simulink model "c28035pmsmfoc_cla"  (R2021b)
settings: Solver=FixedStepDiscrete  StartTime=0.0  StopTime=inf  RelTol=1e-3  EnableMultiTasking=on
PreLoadFcn:
  | c28035pmsmfoc_data_cla;
model workspace (MAT data in the model file):
  encoderResolution = 2000
  hallOffset = '0.5'
  indexOffset = 850
  polePairs = '4'
values from neighbouring files (symbols this model uses):
  Hall_position_offset = 0.57    [c28027pmsmfoc_data.m]    (also in c28035pmsmfoc_data.m; c28035pmsmfoc_data_cla.m; c28069pmsmfoc_data.m)
  PWM_Counter_Period = CPU_frequency/PWM_frequency/2    (= 1500)    [c28027pmsmfoc_data.m]    (also in c28035pmsmfoc_data.m; c28035pmsmfoc_data_cla.m = 2500; c28069pmsmfoc_data.m = 2250)
  Speed_per_unit_scaler = 1200    [c28027pmsmfoc_data.m]    (also in c28035pmsmfoc_data.m; c28035pmsmfoc_data_cla.m = 600; c28069pmsmfoc_data.m)
  Speed_rpm_scaler = 60*CPU_frequency/Pole_pairs/2    (= 450000000)    [c28027pmsmfoc_data.m]    (also in c28035pmsmfoc_data.m; c28035pmsmfoc_data_cla.m; c28069pmsmfoc_data.m = 675000000)
undefined symbols (not defined in the file or in its folder): codertarget, Down, GPTRIP1SEL, GPTRIP2SEL, TZ1, TZ2, Up
libraries: idelinklib_common x16, tiiqmathlib x7, hall_sensor_lib x7, c2802xlib x6, simulink x3, c2803xlib x2, etargetslib x2, demo_controls x1, c2806xlib x1, c280xlib x1, c2000lib x1
(part 3 of 3)

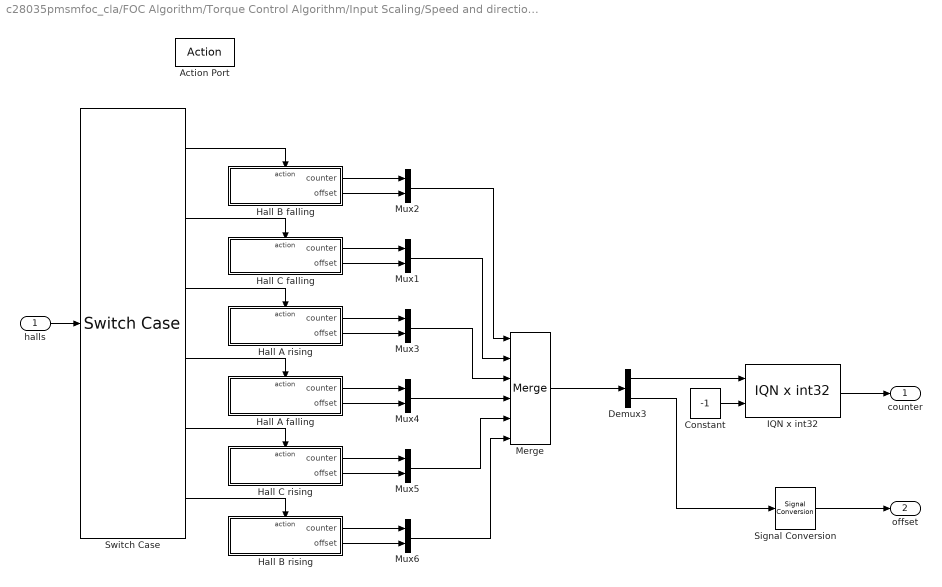
== system c28035pmsmfoc_cla/FOC Algorithm/Torque Control Algorithm/Input Scaling/Speed and direction are valid Use speed to extrapolate position/Extract Position from Halls/Direction 1 Provides offset and counter values ==
  halls : Inport
  Action Port : ActionPort  ActionPortLabel=if(u1 ~= 0)
  Constant : Constant  Value=-1  OutDataTypeStr=int32
  Demux3 : Demux  Outputs=2
  Hall A falling : Subsystem  TreatAsAtomicUnit=on
  Hall A rising : Subsystem  TreatAsAtomicUnit=on
  Hall B falling : Subsystem  TreatAsAtomicUnit=on
  Hall B rising : Subsystem  TreatAsAtomicUnit=on
  Hall C falling : Subsystem  TreatAsAtomicUnit=on
  Hall C rising : Subsystem  TreatAsAtomicUnit=on
  IQN x int32 : tiiqmathlib/IQN x int32
      settings: SourceProductBaseCode=TIC2000
  Merge : Merge  Inputs=6
  Mux{1..6} (6 alike) : Mux  Inputs=2
  Signal Conversion : SignalConversion  OverrideOpt=on
  Switch Case : SwitchCase  CaseConditions={1,2,3,4,5,6}  ShowDefaultCase=off
  counter : Outport
  offset : Outport  Port=2
  wires:
  Hall B falling/1(counter) -> Mux2/1
  Hall B falling/2(offset) -> Mux2/2
  Hall C falling/1(counter) -> Mux1/1
  Hall C falling/2(offset) -> Mux1/2
  Hall A rising/1(counter) -> Mux3/1
  Hall A rising/2(offset) -> Mux3/2
  Hall A falling/1(counter) -> Mux4/1
  Hall A falling/2(offset) -> Mux4/2
  Hall C rising/1(counter) -> Mux5/1
  Hall C rising/2(offset) -> Mux5/2
  Hall B rising/1(counter) -> Mux6/1
  Hall B rising/2(offset) -> Mux6/2
  Mux2/1 -> Merge/1
  Mux1/1 -> Merge/2
  Mux3/1 -> Merge/3
  Mux4/1 -> Merge/4
  Mux5/1 -> Merge/5
  Mux6/1 -> Merge/6
  Merge/1 -> Demux3/1
  Demux3/1 -> IQN x int32/1
  Demux3/2 -> Signal Conversion/1
  IQN x int32/1 -> counter/1
  Constant/1 -> IQN x int32/2
  halls/1 -> Switch Case/1
  Switch Case/2 -> Hall C falling/Action
  Switch Case/5 -> Hall C rising/Action
  Switch Case/6 -> Hall B rising/Action
  Switch Case/1 -> Hall B falling/Action
  Switch Case/3 -> Hall A rising/Action
  Switch Case/4 -> Hall A falling/Action
  Signal Conversion/1 -> offset/1

== system c28035pmsmfoc_cla/FOC Algorithm/Torque Control Algorithm/Generating Space Vectors/Generating Raw Space Vectors/SVGen/Sectors 1//2//3/Sector 1 ==
  Vb* : Inport
  Vc* : Inport  Port=2
  Action Port : ActionPort  ActionPortLabel=else
  Add : Sum  Inputs=--+
  Add1 : Sum
  Add2 : Sum
  Constant : Constant  OutDataTypeStr=Inherit: Inherit via back propagation
  Constant1 : Constant  Value=0.5  OutDataTypeStr=Inherit: Inherit via back propagation
  Product : Product
  Signal Conversion : SignalConversion  OverrideOpt=off
  Signal Conversion1 : SignalConversion  OverrideOpt=off
  Ta* : Outport
  Tb* : Outport  Port=2
  Tc* : Outport  Port=3
  wires:
  Add1/1 -> Tc*/1
  Vc*/1 -> Add2/1, Add/2
  Vb*/1 -> Add1/2, Add/1
  Add2/1 -> Signal Conversion1/1, Add1/1
  Constant1/1 -> Product/2
  Add/1 -> Product/1
  Product/1 -> Signal Conversion/1, Add2/2
  Constant/1 -> Add/3
  Signal Conversion/1 -> Tb*/1
  Signal Conversion1/1 -> Ta*/1

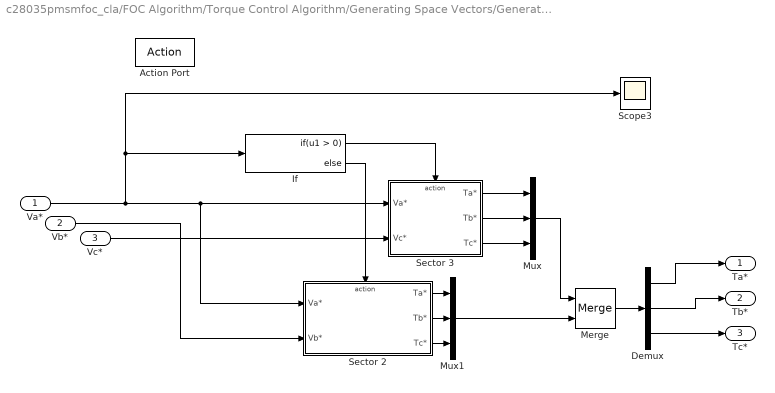
== system c28035pmsmfoc_cla/FOC Algorithm/Torque Control Algorithm/Generating Space Vectors/Generating Raw Space Vectors/SVGen/Sectors 1//2//3/Sector 2 and 3 ==
  Va* : Inport
  Vb* : Inport  Port=2
  Vc* : Inport  Port=3
  Action Port : ActionPort  ActionPortLabel=if(u1 > 0)
  Demux : Demux  Outputs=3
  If : If
  Merge : Merge
  Mux : Mux  Inputs=3
  Mux1 : Mux  Inputs=3
  Scope3 : Scope
  Sector 2 : Subsystem  TreatAsAtomicUnit=on
  Sector 3 : Subsystem  TreatAsAtomicUnit=on
  Ta* : Outport
  Tb* : Outport  Port=2
  Tc* : Outport  Port=3
  wires:
  Va*/1 -> Sector 2/1(Va*), Sector 3/1(Va*), If/1, Scope3/1
  Vb*/1 -> Sector 2/2(Vb*)
  If/1 -> Sector 3/Action
  If/2 -> Sector 2/Action
  Vc*/1 -> Sector 3/2(Vc*)
  Sector 3/1(Ta*) -> Mux/1
  Sector 3/2(Tb*) -> Mux/2
  Sector 3/3(Tc*) -> Mux/3
  Sector 2/1(Ta*) -> Mux1/1
  Sector 2/2(Tb*) -> Mux1/2
  Sector 2/3(Tc*) -> Mux1/3
  Mux/1 -> Merge/1
  Mux1/1 -> Merge/2
  Merge/1 -> Demux/1
  Demux/1 -> Ta*/1
  Demux/2 -> Tb*/1
  Demux/3 -> Tc*/1

== system c28035pmsmfoc_cla/FOC Algorithm/Torque Control Algorithm/Generating Space Vectors/Generating Raw Space Vectors/SVGen/Sectors 4//5//6/Sector 4 and 5 ==
  Va* : Inport
  Vb* : Inport  Port=2
  Vc* : Inport  Port=3
  Action Port : ActionPort  ActionPortLabel=else
  Demux : Demux  Outputs=3
  If : If
  Merge : Merge
  Mux : Mux  Inputs=3
  Mux1 : Mux  Inputs=3
  Sector 4 : Subsystem  TreatAsAtomicUnit=on
  Sector 5 : Subsystem  TreatAsAtomicUnit=on
  Ta* : Outport
  Tb* : Outport  Port=2
  Tc* : Outport  Port=3
  wires:
  Va*/1 -> If/1, Sector 4/1(Va*), Sector 5/1(Va*)
  Demux/3 -> Tc*/1
  Demux/2 -> Tb*/1
  Demux/1 -> Ta*/1
  Merge/1 -> Demux/1
  Mux1/1 -> Merge/2
  Mux/1 -> Merge/1
  Sector 4/3(Tc*) -> Mux1/3
  Sector 4/2(Tb*) -> Mux1/2
  Sector 4/1(Ta*) -> Mux1/1
  Sector 5/3(Tc*) -> Mux/3
  Sector 5/2(Tb*) -> Mux/2
  Sector 5/1(Ta*) -> Mux/1
  Vc*/1 -> Sector 4/2(Vc*)
  Vb*/1 -> Sector 5/2(Vb*)
  If/2 -> Sector 4/Action
  If/1 -> Sector 5/Action

== system c28035pmsmfoc_cla/FOC Algorithm/Torque Control Algorithm/Generating Space Vectors/Generating Raw Space Vectors/SVGen/Sectors 4//5//6/Sector 6 ==
  Vb* : Inport
  Vc* : Inport  Port=2
  Action Port : ActionPort  ActionPortLabel=if(u1 > 0)
  Add : Sum  Inputs=+++
  Add1 : Sum  Inputs=+-
  Add2 : Sum  Inputs=-+
  Constant : Constant  OutDataTypeStr=Inherit: Inherit via back propagation
  Constant1 : Constant  Value=0.5  OutDataTypeStr=Inherit: Inherit via back propagation
  Product : Product
  Signal Conversion1 : SignalConversion  OverrideOpt=off
  Signal Conversion2 : SignalConversion  OverrideOpt=off
  Ta* : Outport
  Tb* : Outport  Port=2
  Tc* : Outport  Port=3
  wires:
  Add1/1 -> Tb*/1
  Add2/1 -> Add1/1, Signal Conversion2/1
  Constant1/1 -> Product/2
  Add/1 -> Product/1
  Product/1 -> Add2/2, Signal Conversion1/1
  Constant/1 -> Add/3
  Vc*/1 -> Add1/2, Add/2
  Vb*/1 -> Add2/1, Add/1
  Signal Conversion2/1 -> Ta*/1
  Signal Conversion1/1 -> Tc*/1

== system c28035pmsmfoc_cla/FOC Algorithm/Torque Control Algorithm/Generating Space Vectors/Generating Raw Space Vectors/control/PID Controller/UD_REG3 ==
  up_reg3 : Inport
  PrevOut : Inport  Port=2
  Constant : Constant  Value=derivativeGain  OutDataTypeStr=Inherit: Inherit via back propagation
  Product : Product  OutDataTypeStr=Inherit: Same as first input
  Sum2 : Sum  Inputs=+-
  Out1 : Outport
  wires:
  Constant/1 -> Product/1
  Product/1 -> Out1/1
  Sum2/1 -> Product/2
  PrevOut/1 -> Sum2/2
  up_reg3/1 -> Sum2/1

== system c28035pmsmfoc_cla/FOC Algorithm/Torque Control Algorithm/Generating Space Vectors/Generating Raw Space Vectors/control/PID Controller/UI_REG3 ==
  OLD_UI_REG3 : Inport
  up_reg3 : Inport  Port=2
  saterr_reg3 : Inport  Port=3
  Constant : Constant  Value=integralGain  OutDataTypeStr=Inherit: Inherit via back propagation
  Constant1 : Constant  Value=correctionGain  OutDataTypeStr=Inherit: Inherit via back propagation
  Product : Product  OutDataTypeStr=Inherit: Same as first input
  Product1 : Product  OutDataTypeStr=Inherit: Same as first input
  Sum1 : Sum  Inputs=+++
  UI_REG1 : Outport
  wires:
  Constant1/1 -> Product1/1
  saterr_reg3/1 -> Product1/2
  Constant/1 -> Product/1
  up_reg3/1 -> Product/2
  Sum1/1 -> UI_REG1/1
  Product1/1 -> Sum1/3
  Product/1 -> Sum1/2
  OLD_UI_REG3/1 -> Sum1/1

== system c28035pmsmfoc_cla/FOC Algorithm/Torque Control Algorithm/Generating Space Vectors/Generating Raw Space Vectors/control/PID Controller1/UD_REG3 ==
  up_reg3 : Inport
  PrevOut : Inport  Port=2
  Constant : Constant  Value=derivativeGain  OutDataTypeStr=Inherit: Inherit via back propagation
  Product : Product  OutDataTypeStr=Inherit: Same as first input
  Sum2 : Sum  Inputs=+-
  Out1 : Outport
  wires:
  Constant/1 -> Product/1
  Product/1 -> Out1/1
  Sum2/1 -> Product/2
  PrevOut/1 -> Sum2/2
  up_reg3/1 -> Sum2/1

== system c28035pmsmfoc_cla/FOC Algorithm/Torque Control Algorithm/Generating Space Vectors/Generating Raw Space Vectors/control/PID Controller1/UI_REG3 ==
  OLD_UI_REG3 : Inport
  up_reg3 : Inport  Port=2
  saterr_reg3 : Inport  Port=3
  Constant : Constant  Value=integralGain  OutDataTypeStr=Inherit: Inherit via back propagation
  Constant1 : Constant  Value=correctionGain  OutDataTypeStr=Inherit: Inherit via back propagation
  Product : Product  OutDataTypeStr=Inherit: Same as first input
  Product1 : Product  OutDataTypeStr=Inherit: Same as first input
  Sum1 : Sum  Inputs=+++
  UI_REG1 : Outport
  wires:
  Constant1/1 -> Product1/1
  saterr_reg3/1 -> Product1/2
  Constant/1 -> Product/1
  up_reg3/1 -> Product/2
  Sum1/1 -> UI_REG1/1
  Product1/1 -> Sum1/3
  Product/1 -> Sum1/2
  OLD_UI_REG3/1 -> Sum1/1

== system c28035pmsmfoc_cla/FOC Algorithm/Torque Control Algorithm/Input Scaling/Speed and direction are valid Use speed to extrapolate position/Extract Position from Halls/Direction 0 Provides offset and counter values/Hall A falling ==
  Action Port : ActionPort  ActionPortLabel=case [ 2 ]:
  Constant : Constant  Value=1/2  OutDataTypeStr=fixdt(1,32,17)
  Data Type Conversion1 : DataTypeConversion  OutDataTypeStr=fixdt(1,32,17)  ConvertRealWorld=Stored Integer (SI)
  ECap1Regs.TSCTR1 : idelinklib_common/Memory Copy  copyFrom=Specified source code symbol  copyFromAddressSource=Specify via dialog  copyFromAddress=hex2dec('00001000')  copyFromSrcCode=&ECap1Regs.TSCTR  dataTypeFrom=uint32  dataDimensionFrom=1  useOffsetFrom=off  offsetFromSrc=Specify via dialog  offsetFrom=0  strideFrom=1  copyTo=Output port  copyToAddressSource=Specify via dialog  copyToAddress=hex2dec('00002000')  copyToSrcCode=myVariableDst  dataTypeTo=uint32  useOffsetTo=off  offsetToSrc=Specify via dialog  offsetTo=0  strideTo=1  sampleTime=-1  useInitValue=off  initValueSrc=Specify constant value  initValue=1  initValueSrcCode=myInitValueVariable  useAsMask=off  maskOperator=bitwise AND  useTermValue=off  termValue=1  isRealtimeEnabled=off  emitCCBeforeWrite=off  CCBeforeWrite=/* Custom Code Before Write*/  emitCCAfterWrite=off  CCAfterWrite=/* Custom Code After Write*/  useDMACopy=off  enableBlockingMode=off
      settings: SourceProductBaseCode=ME
  counter : Outport
  offset : Outport  Port=2
  wires:
  Constant/1 -> offset/1
  ECap1Regs.TSCTR1/1 -> Data Type Conversion1/1
  Data Type Conversion1/1 -> counter/1

== system c28035pmsmfoc_cla/FOC Algorithm/Torque Control Algorithm/Input Scaling/Speed and direction are valid Use speed to extrapolate position/Extract Position from Halls/Direction 0 Provides offset and counter values/Hall A rising ==
  Action Port : ActionPort  ActionPortLabel=case [ 5 ]:
  Constant : Constant  Value=0  OutDataTypeStr=fixdt(1,32,17)
  Data Type Conversion1 : DataTypeConversion  OutDataTypeStr=fixdt(1,32,17)  ConvertRealWorld=Stored Integer (SI)
  ECap1Regs.TSCTR1 : idelinklib_common/Memory Copy  copyFrom=Specified source code symbol  copyFromAddressSource=Specify via dialog  copyFromAddress=hex2dec('00001000')  copyFromSrcCode=&ECap1Regs.TSCTR  dataTypeFrom=uint32  dataDimensionFrom=1  useOffsetFrom=off  offsetFromSrc=Specify via dialog  offsetFrom=0  strideFrom=1  copyTo=Output port  copyToAddressSource=Specify via dialog  copyToAddress=hex2dec('00002000')  copyToSrcCode=myVariableDst  dataTypeTo=uint32  useOffsetTo=off  offsetToSrc=Specify via dialog  offsetTo=0  strideTo=1  sampleTime=-1  useInitValue=off  initValueSrc=Specify constant value  initValue=1  initValueSrcCode=myInitValueVariable  useAsMask=off  maskOperator=bitwise AND  useTermValue=off  termValue=1  isRealtimeEnabled=off  emitCCBeforeWrite=off  CCBeforeWrite=/* Custom Code Before Write*/  emitCCAfterWrite=off  CCAfterWrite=/* Custom Code After Write*/  useDMACopy=off  enableBlockingMode=off
      settings: SourceProductBaseCode=ME
  counter : Outport
  offset : Outport  Port=2
  wires:
  Constant/1 -> offset/1
  ECap1Regs.TSCTR1/1 -> Data Type Conversion1/1
  Data Type Conversion1/1 -> counter/1

== system c28035pmsmfoc_cla/FOC Algorithm/Torque Control Algorithm/Input Scaling/Speed and direction are valid Use speed to extrapolate position/Extract Position from Halls/Direction 0 Provides offset and counter values/Hall B falling ==
  Action Port : ActionPort  ActionPortLabel=case [ 4 ]:
  Add : Sum  Inputs=-+  OutDataTypeStr=Inherit: Same as first input
  Constant : Constant  Value=5/6  OutDataTypeStr=fixdt(1,32,17)
  Data Store Read : DataStoreRead  DataStoreName=ECap1_counter_XINT1_latch  IndexOptions=Index vector (dialog)  Indices=1  OutputSizes=1
  Data Type Conversion1 : DataTypeConversion  OutDataTypeStr=fixdt(1,32,17)  ConvertRealWorld=Stored Integer (SI)
  ECap1Regs.TSCTR : idelinklib_common/Memory Copy  copyFrom=Specified source code symbol  copyFromAddressSource=Specify via dialog  copyFromAddress=hex2dec('00001000')  copyFromSrcCode=&ECap1Regs.TSCTR  dataTypeFrom=uint32  dataDimensionFrom=1  useOffsetFrom=off  offsetFromSrc=Specify via dialog  offsetFrom=0  strideFrom=1  copyTo=Output port  copyToAddressSource=Specify via dialog  copyToAddress=hex2dec('00002000')  copyToSrcCode=myVariableDst  dataTypeTo=uint32  useOffsetTo=off  offsetToSrc=Specify via dialog  offsetTo=0  strideTo=1  sampleTime=-1  useInitValue=off  initValueSrc=Specify constant value  initValue=1  initValueSrcCode=myInitValueVariable  useAsMask=off  maskOperator=bitwise AND  useTermValue=off  termValue=1  isRealtimeEnabled=off  emitCCBeforeWrite=off  CCBeforeWrite=/* Custom Code Before Write*/  emitCCAfterWrite=off  CCAfterWrite=/* Custom Code After Write*/  useDMACopy=off  enableBlockingMode=off
      settings: SourceProductBaseCode=ME
  counter : Outport
  offset : Outport  Port=2
  wires:
  Constant/1 -> offset/1
  Data Type Conversion1/1 -> counter/1
  Data Store Read/1 -> Add/1
  ECap1Regs.TSCTR/1 -> Add/2
  Add/1 -> Data Type Conversion1/1

== system c28035pmsmfoc_cla/FOC Algorithm/Torque Control Algorithm/Input Scaling/Speed and direction are valid Use speed to extrapolate position/Extract Position from Halls/Direction 0 Provides offset and counter values/Hall B rising ==
  Action Port : ActionPort  ActionPortLabel=case [ 3 ]:
  Add : Sum  Inputs=-+  OutDataTypeStr=Inherit: Same as first input
  Constant : Constant  Value=2/6  OutDataTypeStr=fixdt(1,32,17)
  Data Store Read : DataStoreRead  DataStoreName=ECap1_counter_XINT1_latch  IndexOptions=Index vector (dialog)  Indices=1  OutputSizes=1
  Data Type Conversion1 : DataTypeConversion  OutDataTypeStr=fixdt(1,32,17)  ConvertRealWorld=Stored Integer (SI)
  ECap1Regs.TSCTR : idelinklib_common/Memory Copy  copyFrom=Specified source code symbol  copyFromAddressSource=Specify via dialog  copyFromAddress=hex2dec('00001000')  copyFromSrcCode=&ECap1Regs.TSCTR  dataTypeFrom=uint32  dataDimensionFrom=1  useOffsetFrom=off  offsetFromSrc=Specify via dialog  offsetFrom=0  strideFrom=1  copyTo=Output port  copyToAddressSource=Specify via dialog  copyToAddress=hex2dec('00002000')  copyToSrcCode=myVariableDst  dataTypeTo=uint32  useOffsetTo=off  offsetToSrc=Specify via dialog  offsetTo=0  strideTo=1  sampleTime=-1  useInitValue=off  initValueSrc=Specify constant value  initValue=1  initValueSrcCode=myInitValueVariable  useAsMask=off  maskOperator=bitwise AND  useTermValue=off  termValue=1  isRealtimeEnabled=off  emitCCBeforeWrite=off  CCBeforeWrite=/* Custom Code Before Write*/  emitCCAfterWrite=off  CCAfterWrite=/* Custom Code After Write*/  useDMACopy=off  enableBlockingMode=off
      settings: SourceProductBaseCode=ME
  counter : Outport
  offset : Outport  Port=2
  wires:
  Constant/1 -> offset/1
  Data Type Conversion1/1 -> counter/1
  Data Store Read/1 -> Add/1
  ECap1Regs.TSCTR/1 -> Add/2
  Add/1 -> Data Type Conversion1/1

== system c28035pmsmfoc_cla/FOC Algorithm/Torque Control Algorithm/Input Scaling/Speed and direction are valid Use speed to extrapolate position/Extract Position from Halls/Direction 0 Provides offset and counter values/Hall C falling ==
  Action Port : ActionPort  ActionPortLabel=case [ 1 ]:
  Add : Sum  Inputs=-+  OutDataTypeStr=Inherit: Same as first input
  Constant : Constant  Value=1/6  OutDataTypeStr=fixdt(1,32,17)
  Data Store Read : DataStoreRead  DataStoreName=ECap1_counter_XINT2_latch  IndexOptions=Index vector (dialog)  Indices=1  OutputSizes=1
  Data Type Conversion1 : DataTypeConversion  OutDataTypeStr=fixdt(1,32,17)  ConvertRealWorld=Stored Integer (SI)
  ECap1Regs.TSCTR : idelinklib_common/Memory Copy  copyFrom=Specified source code symbol  copyFromAddressSource=Specify via dialog  copyFromAddress=hex2dec('00001000')  copyFromSrcCode=&ECap1Regs.TSCTR  dataTypeFrom=uint32  dataDimensionFrom=1  useOffsetFrom=off  offsetFromSrc=Specify via dialog  offsetFrom=0  strideFrom=1  copyTo=Output port  copyToAddressSource=Specify via dialog  copyToAddress=hex2dec('00002000')  copyToSrcCode=myVariableDst  dataTypeTo=uint32  useOffsetTo=off  offsetToSrc=Specify via dialog  offsetTo=0  strideTo=1  sampleTime=-1  useInitValue=off  initValueSrc=Specify constant value  initValue=1  initValueSrcCode=myInitValueVariable  useAsMask=off  maskOperator=bitwise AND  useTermValue=off  termValue=1  isRealtimeEnabled=off  emitCCBeforeWrite=off  CCBeforeWrite=/* Custom Code Before Write*/  emitCCAfterWrite=off  CCAfterWrite=/* Custom Code After Write*/  useDMACopy=off  enableBlockingMode=off
      settings: SourceProductBaseCode=ME
  counter : Outport
  offset : Outport  Port=2
  wires:
  Constant/1 -> offset/1
  Data Type Conversion1/1 -> counter/1
  Data Store Read/1 -> Add/1
  ECap1Regs.TSCTR/1 -> Add/2
  Add/1 -> Data Type Conversion1/1

== system c28035pmsmfoc_cla/FOC Algorithm/Torque Control Algorithm/Input Scaling/Speed and direction are valid Use speed to extrapolate position/Extract Position from Halls/Direction 0 Provides offset and counter values/Hall C rising ==
  Action Port : ActionPort  ActionPortLabel=case [ 6 ]:
  Add : Sum  Inputs=-+  OutDataTypeStr=Inherit: Same as first input
  Constant : Constant  Value=2/3  OutDataTypeStr=fixdt(1,32,17)
  Data Store Read : DataStoreRead  DataStoreName=ECap1_counter_XINT2_latch  IndexOptions=Index vector (dialog)  Indices=1  OutputSizes=1
  Data Type Conversion1 : DataTypeConversion  OutDataTypeStr=fixdt(1,32,17)  ConvertRealWorld=Stored Integer (SI)
  ECap1Regs.TSCTR : idelinklib_common/Memory Copy  copyFrom=Specified source code symbol  copyFromAddressSource=Specify via dialog  copyFromAddress=hex2dec('00001000')  copyFromSrcCode=&ECap1Regs.TSCTR  dataTypeFrom=uint32  dataDimensionFrom=1  useOffsetFrom=off  offsetFromSrc=Specify via dialog  offsetFrom=0  strideFrom=1  copyTo=Output port  copyToAddressSource=Specify via dialog  copyToAddress=hex2dec('00002000')  copyToSrcCode=myVariableDst  dataTypeTo=uint32  useOffsetTo=off  offsetToSrc=Specify via dialog  offsetTo=0  strideTo=1  sampleTime=-1  useInitValue=off  initValueSrc=Specify constant value  initValue=1  initValueSrcCode=myInitValueVariable  useAsMask=off  maskOperator=bitwise AND  useTermValue=off  termValue=1  isRealtimeEnabled=off  emitCCBeforeWrite=off  CCBeforeWrite=/* Custom Code Before Write*/  emitCCAfterWrite=off  CCAfterWrite=/* Custom Code After Write*/  useDMACopy=off  enableBlockingMode=off
      settings: SourceProductBaseCode=ME
  counter : Outport
  offset : Outport  Port=2
  wires:
  Constant/1 -> offset/1
  Data Type Conversion1/1 -> counter/1
  Data Store Read/1 -> Add/1
  ECap1Regs.TSCTR/1 -> Add/2
  Add/1 -> Data Type Conversion1/1

== system c28035pmsmfoc_cla/FOC Algorithm/Torque Control Algorithm/Input Scaling/Speed and direction are valid Use speed to extrapolate position/Extract Position from Halls/Direction 1 Provides offset and counter values/Hall A falling ==
  Action Port : ActionPort  ActionPortLabel=case [ 4 ]:
  Constant : Constant  OutDataTypeStr=fixdt(1,32,17)
  Data Type Conversion1 : DataTypeConversion  OutDataTypeStr=fixdt(1,32,17)  ConvertRealWorld=Stored Integer (SI)
  ECap1Regs.TSCTR1 : idelinklib_common/Memory Copy  copyFrom=Specified source code symbol  copyFromAddressSource=Specify via dialog  copyFromAddress=hex2dec('00001000')  copyFromSrcCode=&ECap1Regs.TSCTR  dataTypeFrom=uint32  dataDimensionFrom=1  useOffsetFrom=off  offsetFromSrc=Specify via dialog  offsetFrom=0  strideFrom=1  copyTo=Output port  copyToAddressSource=Specify via dialog  copyToAddress=hex2dec('00002000')  copyToSrcCode=myVariableDst  dataTypeTo=uint32  useOffsetTo=off  offsetToSrc=Specify via dialog  offsetTo=0  strideTo=1  sampleTime=-1  useInitValue=off  initValueSrc=Specify constant value  initValue=1  initValueSrcCode=myInitValueVariable  useAsMask=off  maskOperator=bitwise AND  useTermValue=off  termValue=1  isRealtimeEnabled=off  emitCCBeforeWrite=off  CCBeforeWrite=/* Custom Code Before Write*/  emitCCAfterWrite=off  CCAfterWrite=/* Custom Code After Write*/  useDMACopy=off  enableBlockingMode=off
      settings: SourceProductBaseCode=ME
  counter : Outport
  offset : Outport  Port=2
  wires:
  Data Type Conversion1/1 -> counter/1
  ECap1Regs.TSCTR1/1 -> Data Type Conversion1/1
  Constant/1 -> offset/1

== system c28035pmsmfoc_cla/FOC Algorithm/Torque Control Algorithm/Input Scaling/Speed and direction are valid Use speed to extrapolate position/Extract Position from Halls/Direction 1 Provides offset and counter values/Hall A rising ==
  Action Port : ActionPort  ActionPortLabel=case [ 3 ]:
  Constant : Constant  Value=1/2  OutDataTypeStr=fixdt(1,32,17)
  Data Type Conversion1 : DataTypeConversion  OutDataTypeStr=fixdt(1,32,17)  ConvertRealWorld=Stored Integer (SI)
  ECap1Regs.TSCTR1 : idelinklib_common/Memory Copy  copyFrom=Specified source code symbol  copyFromAddressSource=Specify via dialog  copyFromAddress=hex2dec('00001000')  copyFromSrcCode=&ECap1Regs.TSCTR  dataTypeFrom=uint32  dataDimensionFrom=1  useOffsetFrom=off  offsetFromSrc=Specify via dialog  offsetFrom=0  strideFrom=1  copyTo=Output port  copyToAddressSource=Specify via dialog  copyToAddress=hex2dec('00002000')  copyToSrcCode=myVariableDst  dataTypeTo=uint32  useOffsetTo=off  offsetToSrc=Specify via dialog  offsetTo=0  strideTo=1  sampleTime=-1  useInitValue=off  initValueSrc=Specify constant value  initValue=1  initValueSrcCode=myInitValueVariable  useAsMask=off  maskOperator=bitwise AND  useTermValue=off  termValue=1  isRealtimeEnabled=off  emitCCBeforeWrite=off  CCBeforeWrite=/* Custom Code Before Write*/  emitCCAfterWrite=off  CCAfterWrite=/* Custom Code After Write*/  useDMACopy=off  enableBlockingMode=off
      settings: SourceProductBaseCode=ME
  counter : Outport
  offset : Outport  Port=2
  wires:
  Data Type Conversion1/1 -> counter/1
  ECap1Regs.TSCTR1/1 -> Data Type Conversion1/1
  Constant/1 -> offset/1

== system c28035pmsmfoc_cla/FOC Algorithm/Torque Control Algorithm/Input Scaling/Speed and direction are valid Use speed to extrapolate position/Extract Position from Halls/Direction 1 Provides offset and counter values/Hall B falling ==
  Action Port : ActionPort  ActionPortLabel=case [ 1 ]:
  Add : Sum  Inputs=+-  OutDataTypeStr=Inherit: Same as first input
  Constant : Constant  Value=1/3  OutDataTypeStr=fixdt(1,32,17)
  Data Store Read : DataStoreRead  DataStoreName=ECap1_counter_XINT1_latch  IndexOptions=Index vector (dialog)  Indices=1  OutputSizes=1
  Data Type Conversion1 : DataTypeConversion  OutDataTypeStr=fixdt(1,32,17)  ConvertRealWorld=Stored Integer (SI)
  ECap1Regs.TSCTR : idelinklib_common/Memory Copy  copyFrom=Specified source code symbol  copyFromAddressSource=Specify via dialog  copyFromAddress=hex2dec('00001000')  copyFromSrcCode=&ECap1Regs.TSCTR  dataTypeFrom=uint32  dataDimensionFrom=1  useOffsetFrom=off  offsetFromSrc=Specify via dialog  offsetFrom=0  strideFrom=1  copyTo=Output port  copyToAddressSource=Specify via dialog  copyToAddress=hex2dec('00002000')  copyToSrcCode=myVariableDst  dataTypeTo=uint32  useOffsetTo=off  offsetToSrc=Specify via dialog  offsetTo=0  strideTo=1  sampleTime=-1  useInitValue=off  initValueSrc=Specify constant value  initValue=1  initValueSrcCode=myInitValueVariable  useAsMask=off  maskOperator=bitwise AND  useTermValue=off  termValue=1  isRealtimeEnabled=off  emitCCBeforeWrite=off  CCBeforeWrite=/* Custom Code Before Write*/  emitCCAfterWrite=off  CCAfterWrite=/* Custom Code After Write*/  useDMACopy=off  enableBlockingMode=off
      settings: SourceProductBaseCode=ME
  counter : Outport
  offset : Outport  Port=2
  wires:
  Data Type Conversion1/1 -> counter/1
  Constant/1 -> offset/1
  Add/1 -> Data Type Conversion1/1
  ECap1Regs.TSCTR/1 -> Add/1
  Data Store Read/1 -> Add/2

== system c28035pmsmfoc_cla/FOC Algorithm/Torque Control Algorithm/Input Scaling/Speed and direction are valid Use speed to extrapolate position/Extract Position from Halls/Direction 1 Provides offset and counter values/Hall B rising ==
  Action Port : ActionPort  ActionPortLabel=case [ 6 ]:
  Add : Sum  Inputs=-+  OutDataTypeStr=Inherit: Same as first input
  Constant : Constant  Value=5/6  OutDataTypeStr=fixdt(1,32,17)
  Data Store Read : DataStoreRead  DataStoreName=ECap1_counter_XINT1_latch  IndexOptions=Index vector (dialog)  Indices=1  OutputSizes=1
  Data Type Conversion2 : DataTypeConversion  OutDataTypeStr=fixdt(1,32,17)  ConvertRealWorld=Stored Integer (SI)
  ECap1Regs.TSCTR : idelinklib_common/Memory Copy  copyFrom=Specified source code symbol  copyFromAddressSource=Specify via dialog  copyFromAddress=hex2dec('00001000')  copyFromSrcCode=&ECap1Regs.TSCTR  dataTypeFrom=uint32  dataDimensionFrom=1  useOffsetFrom=off  offsetFromSrc=Specify via dialog  offsetFrom=0  strideFrom=1  copyTo=Output port  copyToAddressSource=Specify via dialog  copyToAddress=hex2dec('00002000')  copyToSrcCode=myVariableDst  dataTypeTo=uint32  useOffsetTo=off  offsetToSrc=Specify via dialog  offsetTo=0  strideTo=1  sampleTime=-1  useInitValue=off  initValueSrc=Specify constant value  initValue=1  initValueSrcCode=myInitValueVariable  useAsMask=off  maskOperator=bitwise AND  useTermValue=off  termValue=1  isRealtimeEnabled=off  emitCCBeforeWrite=off  CCBeforeWrite=/* Custom Code Before Write*/  emitCCAfterWrite=off  CCAfterWrite=/* Custom Code After Write*/  useDMACopy=off  enableBlockingMode=off
      settings: SourceProductBaseCode=ME
  counter : Outport
  offset : Outport  Port=2
  wires:
  Data Type Conversion2/1 -> counter/1
  Constant/1 -> offset/1
  Data Store Read/1 -> Add/1
  ECap1Regs.TSCTR/1 -> Add/2
  Add/1 -> Data Type Conversion2/1

== system c28035pmsmfoc_cla/FOC Algorithm/Torque Control Algorithm/Input Scaling/Speed and direction are valid Use speed to extrapolate position/Extract Position from Halls/Direction 1 Provides offset and counter values/Hall C falling ==
  Action Port : ActionPort  ActionPortLabel=case [ 2 ]:
  Add : Sum  Inputs=-+  OutDataTypeStr=Inherit: Same as first input
  Constant : Constant  Value=2/3  OutDataTypeStr=fixdt(1,32,17)
  Data Store Read : DataStoreRead  DataStoreName=ECap1_counter_XINT2_latch  IndexOptions=Index vector (dialog)  Indices=1  OutputSizes=1
  Data Type Conversion1 : DataTypeConversion  OutDataTypeStr=fixdt(1,32,17)  ConvertRealWorld=Stored Integer (SI)
  ECap1Regs.TSCTR : idelinklib_common/Memory Copy  copyFrom=Specified source code symbol  copyFromAddressSource=Specify via dialog  copyFromAddress=hex2dec('00001000')  copyFromSrcCode=&ECap1Regs.TSCTR  dataTypeFrom=uint32  dataDimensionFrom=1  useOffsetFrom=off  offsetFromSrc=Specify via dialog  offsetFrom=0  strideFrom=1  copyTo=Output port  copyToAddressSource=Specify via dialog  copyToAddress=hex2dec('00002000')  copyToSrcCode=myVariableDst  dataTypeTo=uint32  useOffsetTo=off  offsetToSrc=Specify via dialog  offsetTo=0  strideTo=1  sampleTime=-1  useInitValue=off  initValueSrc=Specify constant value  initValue=1  initValueSrcCode=myInitValueVariable  useAsMask=off  maskOperator=bitwise AND  useTermValue=off  termValue=1  isRealtimeEnabled=off  emitCCBeforeWrite=off  CCBeforeWrite=/* Custom Code Before Write*/  emitCCAfterWrite=off  CCAfterWrite=/* Custom Code After Write*/  useDMACopy=off  enableBlockingMode=off
      settings: SourceProductBaseCode=ME
  counter : Outport
  offset : Outport  Port=2
  wires:
  Data Type Conversion1/1 -> counter/1
  Constant/1 -> offset/1
  Data Store Read/1 -> Add/1
  ECap1Regs.TSCTR/1 -> Add/2
  Add/1 -> Data Type Conversion1/1

== system c28035pmsmfoc_cla/FOC Algorithm/Torque Control Algorithm/Input Scaling/Speed and direction are valid Use speed to extrapolate position/Extract Position from Halls/Direction 1 Provides offset and counter values/Hall C rising ==
  Action Port : ActionPort  ActionPortLabel=case [ 5 ]:
  Add : Sum  Inputs=-+  OutDataTypeStr=Inherit: Same as first input
  Constant : Constant  Value=1/6  OutDataTypeStr=fixdt(1,32,17)
  Data Store Read : DataStoreRead  DataStoreName=ECap1_counter_XINT2_latch  IndexOptions=Index vector (dialog)  Indices=1  OutputSizes=1
  Data Type Conversion1 : DataTypeConversion  OutDataTypeStr=fixdt(1,32,17)  ConvertRealWorld=Stored Integer (SI)
  ECap1Regs.TSCTR : idelinklib_common/Memory Copy  copyFrom=Specified source code symbol  copyFromAddressSource=Specify via dialog  copyFromAddress=hex2dec('00001000')  copyFromSrcCode=&ECap1Regs.TSCTR  dataTypeFrom=uint32  dataDimensionFrom=1  useOffsetFrom=off  offsetFromSrc=Specify via dialog  offsetFrom=0  strideFrom=1  copyTo=Output port  copyToAddressSource=Specify via dialog  copyToAddress=hex2dec('00002000')  copyToSrcCode=myVariableDst  dataTypeTo=uint32  useOffsetTo=off  offsetToSrc=Specify via dialog  offsetTo=0  strideTo=1  sampleTime=-1  useInitValue=off  initValueSrc=Specify constant value  initValue=1  initValueSrcCode=myInitValueVariable  useAsMask=off  maskOperator=bitwise AND  useTermValue=off  termValue=1  isRealtimeEnabled=off  emitCCBeforeWrite=off  CCBeforeWrite=/* Custom Code Before Write*/  emitCCAfterWrite=off  CCAfterWrite=/* Custom Code After Write*/  useDMACopy=off  enableBlockingMode=off
      settings: SourceProductBaseCode=ME
  counter : Outport
  offset : Outport  Port=2
  wires:
  Data Type Conversion1/1 -> counter/1
  Constant/1 -> offset/1
  Data Store Read/1 -> Add/1
  ECap1Regs.TSCTR/1 -> Add/2
  Add/1 -> Data Type Conversion1/1

== system c28035pmsmfoc_cla/FOC Algorithm/Torque Control Algorithm/Generating Space Vectors/Generating Raw Space Vectors/SVGen/Sectors 1//2//3/Sector 2 and 3/Sector 2 ==
  Va* : Inport
  Vb* : Inport  Port=2
  Action Port : ActionPort  ActionPortLabel=else
  Add : Sum  Inputs=+-+
  Add1 : Sum  Inputs=+-
  Add2 : Sum
  Constant : Constant  OutDataTypeStr=Inherit: Inherit via back propagation
  Constant1 : Constant  Value=0.5  OutDataTypeStr=Inherit: Inherit via back propagation
  Product : Product
  Signal Conversion : SignalConversion  OverrideOpt=off
  Signal Conversion1 : SignalConversion  OverrideOpt=off
  Ta* : Outport
  Tb* : Outport  Port=2
  Tc* : Outport  Port=3
  wires:
  Add1/1 -> Tb*/1
  Vb*/1 -> Add2/1, Add/2
  Va*/1 -> Add1/2, Add/1
  Add2/1 -> Signal Conversion/1, Add1/1
  Constant1/1 -> Product/2
  Add/1 -> Product/1
  Product/1 -> Signal Conversion1/1, Add2/2
  Constant/1 -> Add/3
  Signal Conversion/1 -> Tc*/1
  Signal Conversion1/1 -> Ta*/1

== system c28035pmsmfoc_cla/FOC Algorithm/Torque Control Algorithm/Generating Space Vectors/Generating Raw Space Vectors/SVGen/Sectors 1//2//3/Sector 2 and 3/Sector 3 ==
  Va* : Inport
  Vc* : Inport  Port=2
  Action Port : ActionPort  ActionPortLabel=if(u1 > 0)
  Add : Sum  Inputs=-++
  Add1 : Sum
  Add2 : Sum  Inputs=-+
  Constant : Constant  OutDataTypeStr=Inherit: Inherit via back propagation
  Constant1 : Constant  Value=0.5  OutDataTypeStr=Inherit: Inherit via back propagation
  Product : Product
  Signal Conversion : SignalConversion  OverrideOpt=off
  Signal Conversion1 : SignalConversion  OverrideOpt=off
  Ta* : Outport
  Tb* : Outport  Port=2
  Tc* : Outport  Port=3
  wires:
  Add1/1 -> Tc*/1
  Vc*/1 -> Add2/1, Add/2
  Va*/1 -> Add1/2, Add/1
  Add2/1 -> Signal Conversion/1, Add1/1
  Constant1/1 -> Product/2
  Add/1 -> Product/1
  Product/1 -> Signal Conversion1/1, Add2/2
  Constant/1 -> Add/3
  Signal Conversion/1 -> Tb*/1
  Signal Conversion1/1 -> Ta*/1

== system c28035pmsmfoc_cla/FOC Algorithm/Torque Control Algorithm/Generating Space Vectors/Generating Raw Space Vectors/SVGen/Sectors 4//5//6/Sector 4 and 5/Sector 4 ==
  Va* : Inport
  Vc* : Inport  Port=2
  Action Port : ActionPort  ActionPortLabel=else
  Add : Sum  Inputs=+-+
  Add1 : Sum
  Add2 : Sum  Inputs=-+
  Constant : Constant  OutDataTypeStr=Inherit: Inherit via back propagation
  Constant1 : Constant  Value=0.5  OutDataTypeStr=Inherit: Inherit via back propagation
  Product : Product
  Signal Conversion : SignalConversion  OverrideOpt=off
  Signal Conversion1 : SignalConversion  OverrideOpt=off
  Ta* : Outport
  Tb* : Outport  Port=2
  Tc* : Outport  Port=3
  wires:
  Add1/1 -> Ta*/1
  Vc*/1 -> Add1/2, Add/2
  Va*/1 -> Add2/1, Add/1
  Add2/1 -> Signal Conversion/1, Add1/1
  Constant1/1 -> Product/2
  Add/1 -> Product/1
  Product/1 -> Signal Conversion1/1, Add2/2
  Constant/1 -> Add/3
  Signal Conversion/1 -> Tb*/1
  Signal Conversion1/1 -> Tc*/1

== system c28035pmsmfoc_cla/FOC Algorithm/Torque Control Algorithm/Generating Space Vectors/Generating Raw Space Vectors/SVGen/Sectors 4//5//6/Sector 4 and 5/Sector 5 ==
  Va* : Inport
  Vb* : Inport  Port=2
  Action Port : ActionPort  ActionPortLabel=if(u1 > 0)
  Add : Sum  Inputs=-++
  Add1 : Sum  Inputs=+-
  Add2 : Sum
  Constant : Constant  OutDataTypeStr=Inherit: Inherit via back propagation
  Constant1 : Constant  Value=0.5  OutDataTypeStr=Inherit: Inherit via back propagation
  Product : Product
  Signal Conversion1 : SignalConversion  OverrideOpt=off
  Signal Conversion2 : SignalConversion  OverrideOpt=off
  Ta* : Outport
  Tb* : Outport  Port=2
  Tc* : Outport  Port=3
  wires:
  Add1/1 -> Ta*/1
  Vb*/1 -> Add1/2, Add/2
  Va*/1 -> Add2/1, Add/1
  Add2/1 -> Signal Conversion2/1, Add1/1
  Constant1/1 -> Product/2
  Add/1 -> Product/1
  Product/1 -> Signal Conversion1/1, Add2/2
  Constant/1 -> Add/3
  Signal Conversion1/1 -> Tb*/1
  Signal Conversion2/1 -> Tc*/1

== matlab function c28035pmsmfoc_cla/FOC Algorithm/Torque Control Algorithm/Generating Space Vectors/Generating Raw Space Vectors/Park Transformation/MATLAB Function ==
  data: u input; y output
function y = fcn(u)
%#codegen
y = single(0);
if isequal(coder.target,'rtw')  
    y = coder.ceval('CLAcos', u);
else
    y = cos(u);
end

== matlab function c28035pmsmfoc_cla/FOC Algorithm/Torque Control Algorithm/Generating Space Vectors/Generating Raw Space Vectors/Inverse Park Transformation/MATLAB Function ==
  data: u input; y output
function y = fcn(u)
%#codegen
y = single(0);
if isequal(coder.target,'rtw') 
    y = coder.ceval('CLAcos', u);
else
    y = cos(u);
end

== matlab function c28035pmsmfoc_cla/FOC Algorithm/Torque Control Algorithm/Generating Space Vectors/Generating Raw Space Vectors/Inverse Park Transformation/MATLAB Function1 ==
  data: u input; y output
function y = fcn(u)
%#codegen
y = single(0);
if isequal(coder.target,'rtw')  
    y = coder.ceval('CLAsin', u);
else
    y = sin(u);
end

== matlab function c28035pmsmfoc_cla/FOC Algorithm/Torque Control Algorithm/Generating Space Vectors/Generating Raw Space Vectors/Park Transformation/MATLAB Function1 ==
  data: u input; y output
function y = fcn(u)
%#codegen
y = single(0);
if isequal(coder.target,'rtw')  
    y = coder.ceval('CLAsin', u);
else
    y = sin(u);
end
